simulink model "s_cd_ramp"  (R2016b)
(part 18 of 40)

      settings: AttributesFormatString=Latency = %<latency>
      mask Display:
      | port_label('input', 1, 'd');
      | port_label('output', 1, 'q');
      | disp(['Z^-', num2str(latency)]);
  pipeline69 : Subsystem  AncestorBlock=casper_library_delays/pipeline  mask(pipeline){latency=2}
      mask help:
      | An explicitly laid-out delay line to avoid mapping to SRL16s
      | for use in pipelining to help achieve timing closure.
      mask init:
      | pipeline_init(gcb,'latency',latency);
      settings: AttributesFormatString=Latency = %<latency>
      mask Display:
      | port_label('input', 1, 'd');
      | port_label('output', 1, 'q');
      | disp(['Z^-', num2str(latency)]);
  pipeline7 : Subsystem  AncestorBlock=casper_library_delays/pipeline  mask(pipeline){latency=2}
      mask help:
      | An explicitly laid-out delay line to avoid mapping to SRL16s
      | for use in pipelining to help achieve timing closure.
      mask init:
      | pipeline_init(gcb,'latency',latency);
      settings: AttributesFormatString=Latency = %<latency>
      mask Display:
      | port_label('input', 1, 'd');
      | port_label('output', 1, 'q');
      | disp(['Z^-', num2str(latency)]);
  pipeline70 : Subsystem  AncestorBlock=casper_library_delays/pipeline  mask(pipeline){latency=2}
      mask help:
      | An explicitly laid-out delay line to avoid mapping to SRL16s
      | for use in pipelining to help achieve timing closure.
      mask init:
      | pipeline_init(gcb,'latency',latency);
      settings: AttributesFormatString=Latency = %<latency>
      mask Display:
      | port_label('input', 1, 'd');
      | port_label('output', 1, 'q');
      | disp(['Z^-', num2str(latency)]);
  pipeline71 : Subsystem  AncestorBlock=casper_library_delays/pipeline  mask(pipeline){latency=2}
      mask help:
      | An explicitly laid-out delay line to avoid mapping to SRL16s
      | for use in pipelining to help achieve timing closure.
      mask init:
      | pipeline_init(gcb,'latency',latency);
      settings: AttributesFormatString=Latency = %<latency>
      mask Display:
      | port_label('input', 1, 'd');
      | port_label('output', 1, 'q');
      | disp(['Z^-', num2str(latency)]);
  pipeline72 : Subsystem  AncestorBlock=casper_library_delays/pipeline  mask(pipeline){latency=2}
      mask help:
      | An explicitly laid-out delay line to avoid mapping to SRL16s
      | for use in pipelining to help achieve timing closure.
      mask init:
      | pipeline_init(gcb,'latency',latency);
      settings: AttributesFormatString=Latency = %<latency>
      mask Display:
      | port_label('input', 1, 'd');
      | port_label('output', 1, 'q');
      | disp(['Z^-', num2str(latency)]);
  pipeline73 : Subsystem  AncestorBlock=casper_library_delays/pipeline  mask(pipeline){latency=2}
      mask help:
      | An explicitly laid-out delay line to avoid mapping to SRL16s
      | for use in pipelining to help achieve timing closure.
      mask init:
      | pipeline_init(gcb,'latency',latency);
      settings: AttributesFormatString=Latency = %<latency>
      mask Display:
      | port_label('input', 1, 'd');
      | port_label('output', 1, 'q');
      | disp(['Z^-', num2str(latency)]);
  pipeline74 : Subsystem  AncestorBlock=casper_library_delays/pipeline  mask(pipeline){latency=2}
      mask help:
      | An explicitly laid-out delay line to avoid mapping to SRL16s
      | for use in pipelining to help achieve timing closure.
      mask init:
      | pipeline_init(gcb,'latency',latency);
      settings: AttributesFormatString=Latency = %<latency>
      mask Display:
      | port_label('input', 1, 'd');
      | port_label('output', 1, 'q');
      | disp(['Z^-', num2str(latency)]);
  pipeline75 : Subsystem  AncestorBlock=casper_library_delays/pipeline  mask(pipeline){latency=2}
      mask help:
      | An explicitly laid-out delay line to avoid mapping to SRL16s
      | for use in pipelining to help achieve timing closure.
      mask init:
      | pipeline_init(gcb,'latency',latency);
      settings: AttributesFormatString=Latency = %<latency>
      mask Display:
      | port_label('input', 1, 'd');
      | port_label('output', 1, 'q');
      | disp(['Z^-', num2str(latency)]);
  pipeline76 : Subsystem  AncestorBlock=casper_library_delays/pipeline  mask(pipeline){latency=2}
      mask help:
      | An explicitly laid-out delay line to avoid mapping to SRL16s
      | for use in pipelining to help achieve timing closure.
      mask init:
      | pipeline_init(gcb,'latency',latency);
      settings: AttributesFormatString=Latency = %<latency>
      mask Display:
      | port_label('input', 1, 'd');
      | port_label('output', 1, 'q');
      | disp(['Z^-', num2str(latency)]);
  pipeline77 : Subsystem  AncestorBlock=casper_library_delays/pipeline  mask(pipeline){latency=2}
      mask help:
      | An explicitly laid-out delay line to avoid mapping to SRL16s
      | for use in pipelining to help achieve timing closure.
      mask init:
      | pipeline_init(gcb,'latency',latency);
      settings: AttributesFormatString=Latency = %<latency>
      mask Display:
      | port_label('input', 1, 'd');
      | port_label('output', 1, 'q');
      | disp(['Z^-', num2str(latency)]);
  pipeline78 : Subsystem  AncestorBlock=casper_library_delays/pipeline  mask(pipeline){latency=2}
      mask help:
      | An explicitly laid-out delay line to avoid mapping to SRL16s
      | for use in pipelining to help achieve timing closure.
      mask init:
      | pipeline_init(gcb,'latency',latency);
      settings: AttributesFormatString=Latency = %<latency>
      mask Display:
      | port_label('input', 1, 'd');
      | port_label('output', 1, 'q');
      | disp(['Z^-', num2str(latency)]);
  pipeline79 : Subsystem  AncestorBlock=casper_library_delays/pipeline  mask(pipeline){latency=2}
      mask help:
      | An explicitly laid-out delay line to avoid mapping to SRL16s
      | for use in pipelining to help achieve timing closure.
      mask init:
      | pipeline_init(gcb,'latency',latency);
      settings: AttributesFormatString=Latency = %<latency>
      mask Display:
      | port_label('input', 1, 'd');
      | port_label('output', 1, 'q');
      | disp(['Z^-', num2str(latency)]);
  pipeline8 : Subsystem  AncestorBlock=casper_library_delays/pipeline  mask(pipeline){latency=2}
      mask help:
      | An explicitly laid-out delay line to avoid mapping to SRL16s
      | for use in pipelining to help achieve timing closure.
      mask init:
      | pipeline_init(gcb,'latency',latency);
      settings: AttributesFormatString=Latency = %<latency>
      mask Display:
      | port_label('input', 1, 'd');
      | port_label('output', 1, 'q');
      | disp(['Z^-', num2str(latency)]);
  pipeline83 : Subsystem  AncestorBlock=casper_library_delays/pipeline  mask(pipeline){latency=2}
      mask help:
      | An explicitly laid-out delay line to avoid mapping to SRL16s
      | for use in pipelining to help achieve timing closure.
      mask init:
      | pipeline_init(gcb,'latency',latency);
      settings: AttributesFormatString=Latency = %<latency>
      mask Display:
      | port_label('input', 1, 'd');
      | port_label('output', 1, 'q');
      | disp(['Z^-', num2str(latency)]);
  pipeline84 : Subsystem  AncestorBlock=casper_library_delays/pipeline  mask(pipeline){latency=2}
      mask help:
      | An explicitly laid-out delay line to avoid mapping to SRL16s
      | for use in pipelining to help achieve timing closure.
      mask init:
      | pipeline_init(gcb,'latency',latency);
      settings: AttributesFormatString=Latency = %<latency>
      mask Display:
      | port_label('input', 1, 'd');
      | port_label('output', 1, 'q');
      | disp(['Z^-', num2str(latency)]);
  pipeline85 : Subsystem  AncestorBlock=casper_library_delays/pipeline  mask(pipeline){latency=2}
      mask help:
      | An explicitly laid-out delay line to avoid mapping to SRL16s
      | for use in pipelining to help achieve timing closure.
      mask init:
      | pipeline_init(gcb,'latency',latency);
      settings: AttributesFormatString=Latency = %<latency>
      mask Display:
      | port_label('input', 1, 'd');
      | port_label('output', 1, 'q');
      | disp(['Z^-', num2str(latency)]);
  pipeline86 : Subsystem  AncestorBlock=casper_library_delays/pipeline  mask(pipeline){latency=2}
      mask help:
      | An explicitly laid-out delay line to avoid mapping to SRL16s
      | for use in pipelining to help achieve timing closure.
      mask init:
      | pipeline_init(gcb,'latency',latency);
      settings: AttributesFormatString=Latency = %<latency>
      mask Display:
      | port_label('input', 1, 'd');
      | port_label('output', 1, 'q');
      | disp(['Z^-', num2str(latency)]);
  pipeline87 : Subsystem  AncestorBlock=casper_library_delays/pipeline  mask(pipeline){latency=2}
      mask help:
      | An explicitly laid-out delay line to avoid mapping to SRL16s
      | for use in pipelining to help achieve timing closure.
      mask init:
      | pipeline_init(gcb,'latency',latency);
      settings: AttributesFormatString=Latency = %<latency>
      mask Display:
      | port_label('input', 1, 'd');
      | port_label('output', 1, 'q');
      | disp(['Z^-', num2str(latency)]);
  pipeline88 : Subsystem  AncestorBlock=casper_library_delays/pipeline  mask(pipeline){latency=2}
      mask help:
      | An explicitly laid-out delay line to avoid mapping to SRL16s
      | for use in pipelining to help achieve timing closure.
      mask init:
      | pipeline_init(gcb,'latency',latency);
      settings: AttributesFormatString=Latency = %<latency>
      mask Display:
      | port_label('input', 1, 'd');
      | port_label('output', 1, 'q');
      | disp(['Z^-', num2str(latency)]);
  pipeline89 : Subsystem  AncestorBlock=casper_library_delays/pipeline  mask(pipeline){latency=2}
      mask help:
      | An explicitly laid-out delay line to avoid mapping to SRL16s
      | for use in pipelining to help achieve timing closure.
      mask init:
      | pipeline_init(gcb,'latency',latency);
      settings: AttributesFormatString=Latency = %<latency>
      mask Display:
      | port_label('input', 1, 'd');
      | port_label('output', 1, 'q');
      | disp(['Z^-', num2str(latency)]);
  pipeline9 : Subsystem  AncestorBlock=casper_library_delays/pipeline  mask(pipeline){latency=2}
      mask help:
      | An explicitly laid-out delay line to avoid mapping to SRL16s
      | for use in pipelining to help achieve timing closure.
      mask init:
      | pipeline_init(gcb,'latency',latency);
      settings: AttributesFormatString=Latency = %<latency>
      mask Display:
      | port_label('input', 1, 'd');
      | port_label('output', 1, 'q');
      | disp(['Z^-', num2str(latency)]);
  pipeline90 : Subsystem  AncestorBlock=casper_library_delays/pipeline  mask(pipeline){latency=2}
      mask help:
      | An explicitly laid-out delay line to avoid mapping to SRL16s
      | for use in pipelining to help achieve timing closure.
      mask init:
      | pipeline_init(gcb,'latency',latency);
      settings: AttributesFormatString=Latency = %<latency>
      mask Display:
      | port_label('input', 1, 'd');
      | port_label('output', 1, 'q');
      | disp(['Z^-', num2str(latency)]);
  pipeline91 : Subsystem  AncestorBlock=casper_library_delays/pipeline  mask(pipeline){latency=2}
      mask help:
      | An explicitly laid-out delay line to avoid mapping to SRL16s
      | for use in pipelining to help achieve timing closure.
      mask init:
      | pipeline_init(gcb,'latency',latency);
      settings: AttributesFormatString=Latency = %<latency>
      mask Display:
      | port_label('input', 1, 'd');
      | port_label('output', 1, 'q');
      | disp(['Z^-', num2str(latency)]);
  pipeline92 : Subsystem  AncestorBlock=casper_library_delays/pipeline  mask(pipeline){latency=1}
      mask help:
      | An explicitly laid-out delay line to avoid mapping to SRL16s
      | for use in pipelining to help achieve timing closure.
      mask init:
      | pipeline_init(gcb,'latency',latency);
      settings: AttributesFormatString=Latency = %<latency>
      mask Display:
      | port_label('input', 1, 'd');
      | port_label('output', 1, 'q');
      | disp(['Z^-', num2str(latency)]);
  pipeline93 : Subsystem  AncestorBlock=casper_library_delays/pipeline  mask(pipeline){latency=2}
      mask help:
      | An explicitly laid-out delay line to avoid mapping to SRL16s
      | for use in pipelining to help achieve timing closure.
      mask init:
      | pipeline_init(gcb,'latency',latency);
      settings: AttributesFormatString=Latency = %<latency>
      mask Display:
      | port_label('input', 1, 'd');
      | port_label('output', 1, 'q');
      | disp(['Z^-', num2str(latency)]);
  pipeline94 : Subsystem  AncestorBlock=casper_library_delays/pipeline  mask(pipeline){latency=2}
      mask help:
      | An explicitly laid-out delay line to avoid mapping to SRL16s
      | for use in pipelining to help achieve timing closure.
      mask init:
      | pipeline_init(gcb,'latency',latency);
      settings: AttributesFormatString=Latency = %<latency>
      mask Display:
      | port_label('input', 1, 'd');
      | port_label('output', 1, 'q');
      | disp(['Z^-', num2str(latency)]);
  pipeline95 : Subsystem  AncestorBlock=casper_library_delays/pipeline  mask(pipeline){latency=2}
      mask help:
      | An explicitly laid-out delay line to avoid mapping to SRL16s
      | for use in pipelining to help achieve timing closure.
      mask init:
      | pipeline_init(gcb,'latency',latency);
      settings: AttributesFormatString=Latency = %<latency>
      mask Display:
      | port_label('input', 1, 'd');
      | port_label('output', 1, 'q');
      | disp(['Z^-', num2str(latency)]);
  pipeline96 : Subsystem  AncestorBlock=casper_library_delays/pipeline  mask(pipeline){latency=2}
      mask help:
      | An explicitly laid-out delay line to avoid mapping to SRL16s
      | for use in pipelining to help achieve timing closure.
      mask init:
      | pipeline_init(gcb,'latency',latency);
      settings: AttributesFormatString=Latency = %<latency>
      mask Display:
      | port_label('input', 1, 'd');
      | port_label('output', 1, 'q');
      | disp(['Z^-', num2str(latency)]);
  qout : Subsystem  Tag=casper:bitsnap  AncestorBlock=casper_library_scopes/bitfield snapshot  mask(bitsnap){io_names=[d00 d01 d02 d03 d04 d05 d06 d07 dvalid sync], io_widths=[10 10 10 10 10 10 10 10 1 1], io_bps=[0 0 0 0 0 0 0 0 0 0], io_types=[0 0 0 0 0 0 0 0 2 2], show_format=on, snap_storage=bram, snap_dram_dimm=2, snap_dram_clock=250, snap_nsamples=11, snap_data_width=128, snap_offset=off, snap_circap=off, snap_value=off, snap_use_dsp48=off, snap_delay=0, extra_names=[c d], extra_widths=[30 2], extra_bps=[0 0], extra_types=[0 0]}
      mask prompts: io_names "Names [msb...lsb]"; io_widths "Bitwidths [msb...lsb]"; io_bps "Binary pts [msb...lsb]"; io_types "Data types [msb...lsb], ufix=0, fix=1, bool=2"; show_format "Print format string?"; snap_storage "Storage medium"; snap_dram_dimm "DRAM dimm"; snap_dram_clock "DRAM clock rate"; snap_nsamples "Number of Samples (2^?)"; snap_data_width "Data width"; snap_offset "Start delay support"; snap_circap "Circular capture support"; snap_value "Extra value capture support"; snap_use_dsp48 "Use DSP48s to implement counters"; snap_delay "Pre-snapshot delay"; extra_names "Names [msb...lsb]"; extra_widths "Widths [msb...lsb]"; extra_bps "Binary pts [msb...lsb]"; extra_types "Data types [msb...lsb], ufix=0, fix=1, bool=2"
      mask help:
      | A wrapped snapshot block. Allows specification of inputs to a snapblock word so the toolflow can automatically set up the scope.
      | See documentation for snapshot for explanation of parameters.
      mask init:
      | bitsnap_init(gcb);
      settings: AttributesFormatString=snap(10):uf10.0,uf10.0,uf10.0,uf10.0,uf10.0,uf10.0,uf10.0,uf10.0,b,b = 82 bits
      mask TypeOptions snap_storage: bram | dram
      mask Callback snap_storage: bitsnap_callback();
      mask TypeOptions snap_dram_dimm: 1 | 2 | 3 | 4
      mask TypeOptions snap_dram_clock: 200 | 250 | 266 | 300 | 333
      mask TypeOptions snap_data_width: 8 | 16 | 32 | 64 | 128
      mask Callback snap_value: bitsnap_callback();
  rdin_stall : xbsIndex_r4/Counter  cnt_type=Count Limited  cnt_to=1  operation=Up  start_count=0  cnt_by_val=1  arith_type=Unsigned  n_bits=1  bin_pt=0  load_pin=off  rst=off  en=on  explicit_period=on  period=1  use_behavioral_HDL=on  implementation=DSP48  use_rpm=off  dbl_ovrd=off  block_type=counter
  reord_dvalid_delay : xbsIndex_r4/Delay  rst=off  infoeditControl=Selection of Reset will increase slice count due to use of real FFs and instead of SRLs  en=off  latency=1  reg_retiming=on  dbl_ovrd=off  block_type=delay
      settings: infoedit=Hardware notes: A delay line is a chain, each link of which is an SRL16 or SRL32 followed by a flip-flop.
  reord_dvalid_delay2 : xbsIndex_r4/Delay  rst=off  infoeditControl=Selection of Reset will increase slice count due to use of real FFs and instead of SRLs  en=off  latency=3  reg_retiming=on  dbl_ovrd=off  block_type=delay
      settings: infoedit=Hardware notes: A delay line is a chain, each link of which is an SRL16 or SRL32 followed by a flip-flop.
  second : xbsIndex_r4/Delay  rst=off  infoeditControl=Selection of Reset will increase slice count due to use of real FFs and instead of SRLs  en=on  latency=1  reg_retiming=on  dbl_ovrd=off  block_type=delay
      settings: block_version=11.4
  sync_counter_en : Subsystem  Tag=xps:sw_reg  AncestorBlock=xps_library/software_register  mask(swreg){io_dir=From Processor, io_delay=0, sample_period=1, names=reg, bitwidths=1, bin_pts=0, arith_types=2, sim_port=off, show_format=on}
      mask prompts: io_dir "I/O direction"; io_delay "I/O delay"; sample_period "Sample period"; names "Bitfield names [msb...lsb]"; bitwidths "Bitfield widths"; bin_pts "Bitfield binary pts"; arith_types "Bitfield types, ufix=0, fix=1, bool=2"; sim_port "Provide sim input/output?"; show_format "Print format string?"
      mask help: A 32-bit software-accessible register. Can be divided into bitfields of varying widths and types using the fields in the block mask.
      mask init:
      | swreg_init(gcb)
      settings: AttributesFormatString=1input:b = 1 bits
      mask TypeOptions io_dir: To Processor | From Processor
      mask Callback io_dir:
      | mask_enables = get_param(gcb, 'MaskEnables');
      | mask_names = get_param(gcb, 'MaskNames');
      | if strcmp(get_param(gcb, 'io_dir'), 'To Processor'),
      |     mask_enables{ismember(mask_names, 'sample_period')} = 'off';
      | else
      |     mask_enables{ismember(mask_names, 'sample_period')} = 'on';
      | end
      | set_param(gcb, 'MaskEnables', mask_enables);
  sync_counter_rst : Subsystem  Tag=xps:sw_reg  AncestorBlock=xps_library/software_register  mask(swreg){io_dir=From Processor, io_delay=0, sample_period=1, names=reg, bitwidths=1, bin_pts=0, arith_types=2, sim_port=off, show_format=on}
      mask prompts: io_dir "I/O direction"; io_delay "I/O delay"; sample_period "Sample period"; names "Bitfield names [msb...lsb]"; bitwidths "Bitfield widths"; bin_pts "Bitfield binary pts"; arith_types "Bitfield types, ufix=0, fix=1, bool=2"; sim_port "Provide sim input/output?"; show_format "Print format string?"
      mask help: A 32-bit software-accessible register. Can be divided into bitfields of varying widths and types using the fields in the block mask.
      mask init:
      | swreg_init(gcb)
      settings: AttributesFormatString=1input:b = 1 bits
      mask TypeOptions io_dir: To Processor | From Processor
      mask Callback io_dir:
      | mask_enables = get_param(gcb, 'MaskEnables');
      | mask_names = get_param(gcb, 'MaskNames');
      | if strcmp(get_param(gcb, 'io_dir'), 'To Processor'),
      |     mask_enables{ismember(mask_names, 'sample_period')} = 'off';
      | else
      |     mask_enables{ismember(mask_names, 'sample_period')} = 'on';
      | end
      | set_param(gcb, 'MaskEnables', mask_enables);
  sync_delay1 : xbsIndex_r4/Delay  rst=off  infoeditControl=Selection of Reset will increase slice count due to use of real FFs and instead of SRLs  en=off  latency=3  reg_retiming=on  dbl_ovrd=off  block_type=delay
      settings: infoedit=Hardware notes: A delay line is a chain, each link of which is an SRL16 or SRL32 followed by a flip-flop.
  sync_delay2 : xbsIndex_r4/Delay  rst=off  infoeditControl=Selection of Reset will increase slice count due to use of real FFs and instead of SRLs  en=off  latency=3  reg_retiming=on  dbl_ovrd=off  block_type=delay
      settings: infoedit=Hardware notes: A delay line is a chain, each link of which is an SRL16 or SRL32 followed by a flip-flop.
  sync_delay{3..5,7..9} (6 alike) : xbsIndex_r4/Delay  rst=off  infoeditControl=Selection of Reset will increase slice count due to use of real FFs and instead of SRLs  en=off  latency=1  reg_retiming=on  dbl_ovrd=off  block_type=delay
      settings: infoedit=Hardware notes: A delay line is a chain, each link of which is an SRL16 or SRL32 followed by a flip-flop.
  sync_delay6 : xbsIndex_r4/Delay  rst=off  infoeditControl=Selection of Reset will increase slice count due to use of real FFs and instead of SRLs  en=off  latency=3  reg_retiming=on  dbl_ovrd=off  block_type=delay
      settings: infoedit=Hardware notes: A delay line is a chain, each link of which is an SRL16 or SRL32 followed by a flip-flop.
  sync_en_fifo : Subsystem  Tag=xps:sw_reg  AncestorBlock=xps_library/software_register  mask(swreg){io_dir=From Processor, io_delay=0, sample_period=1, names=reg, bitwidths=1, bin_pts=0, arith_types=2, sim_port=off, show_format=on}
      mask prompts: io_dir "I/O direction"; io_delay "I/O delay"; sample_period "Sample period"; names "Bitfield names [msb...lsb]"; bitwidths "Bitfield widths"; bin_pts "Bitfield binary pts"; arith_types "Bitfield types, ufix=0, fix=1, bool=2"; sim_port "Provide sim input/output?"; show_format "Print format string?"
      mask help: A 32-bit software-accessible register. Can be divided into bitfields of varying widths and types using the fields in the block mask.
      mask init:
      | swreg_init(gcb)
      settings: AttributesFormatString=1input:b = 1 bits
      mask TypeOptions io_dir: To Processor | From Processor
      mask Callback io_dir:
      | mask_enables = get_param(gcb, 'MaskEnables');
      | mask_names = get_param(gcb, 'MaskNames');
      | if strcmp(get_param(gcb, 'io_dir'), 'To Processor'),
      |     mask_enables{ismember(mask_names, 'sample_period')} = 'off';
      | else
      |     mask_enables{ismember(mask_names, 'sample_period')} = 'on';
      | end
      | set_param(gcb, 'MaskEnables', mask_enables);
  sync_en_qout : Subsystem  Tag=xps:sw_reg  AncestorBlock=xps_library/software_register  mask(swreg){io_dir=From Processor, io_delay=0, sample_period=1, names=reg, bitwidths=1, bin_pts=0, arith_types=2, sim_port=off, show_format=on}
      mask prompts: io_dir "I/O direction"; io_delay "I/O delay"; sample_period "Sample period"; names "Bitfield names [msb...lsb]"; bitwidths "Bitfield widths"; bin_pts "Bitfield binary pts"; arith_types "Bitfield types, ufix=0, fix=1, bool=2"; sim_port "Provide sim input/output?"; show_format "Print format string?"
      mask help: A 32-bit software-accessible register. Can be divided into bitfields of varying widths and types using the fields in the block mask.
      mask init:
      | swreg_init(gcb)
      settings: AttributesFormatString=1input:b = 1 bits
      mask TypeOptions io_dir: To Processor | From Processor
      mask Callback io_dir:
      | mask_enables = get_param(gcb, 'MaskEnables');
      | mask_names = get_param(gcb, 'MaskNames');
      | if strcmp(get_param(gcb, 'io_dir'), 'To Processor'),
      |     mask_enables{ismember(mask_names, 'sample_period')} = 'off';
      | else
      |     mask_enables{ismember(mask_names, 'sample_period')} = 'on';
      | end
      | set_param(gcb, 'MaskEnables', mask_enables);
  sync_en_reord : Subsystem  Tag=xps:sw_reg  AncestorBlock=xps_library/software_register  mask(swreg){io_dir=From Processor, io_delay=0, sample_period=1, names=reg, bitwidths=1, bin_pts=0, arith_types=2, sim_port=off, show_format=on}
      mask prompts: io_dir "I/O direction"; io_delay "I/O delay"; sample_period "Sample period"; names "Bitfield names [msb...lsb]"; bitwidths "Bitfield widths"; bin_pts "Bitfield binary pts"; arith_types "Bitfield types, ufix=0, fix=1, bool=2"; sim_port "Provide sim input/output?"; show_format "Print format string?"
      mask help: A 32-bit software-accessible register. Can be divided into bitfields of varying widths and types using the fields in the block mask.
      mask init:
      | swreg_init(gcb)
      settings: AttributesFormatString=1input:b = 1 bits
      mask TypeOptions io_dir: To Processor | From Processor
      mask Callback io_dir:
      | mask_enables = get_param(gcb, 'MaskEnables');
      | mask_names = get_param(gcb, 'MaskNames');
      | if strcmp(get_param(gcb, 'io_dir'), 'To Processor'),
      |     mask_enables{ismember(mask_names, 'sample_period')} = 'off';
      | else
      |     mask_enables{ismember(mask_names, 'sample_period')} = 'on';
      | end
      | set_param(gcb, 'MaskEnables', mask_enables);
  tag_stall : xbsIndex_r4/Counter  cnt_type=Count Limited  cnt_to=1  operation=Up  start_count=0  cnt_by_val=1  arith_type=Unsigned  n_bits=1  bin_pt=0  load_pin=off  rst=off  en=on  explicit_period=on  period=1  use_behavioral_HDL=on  implementation=DSP48  use_rpm=off  dbl_ovrd=off  block_type=counter
  wrin_stall : xbsIndex_r4/Counter  cnt_type=Count Limited  cnt_to=1  operation=Up  start_count=0  cnt_by_val=1  arith_type=Unsigned  n_bits=1  bin_pt=0  load_pin=off  rst=off  en=on  explicit_period=on  period=1  use_behavioral_HDL=on  implementation=DSP48  use_rpm=off  dbl_ovrd=off  block_type=counter
  sync_out : Outport
  q : Outport  Port=2
  dv : Outport  Port=3
  hmc_error : Outport  Port=4
  parity_error : Outport  Port=5
  misco : Outport  Port=6
  tag scope: sync_trig=global
  wires:
  Logical6/1 -> Logical7/2, Delay68/1
  Delay44/1 -> Delay66/1, Logical7/1
  Delay37/1 -> Delay36/1, Logical4/2
  Delay31/1 -> Logical6/1
  Delay15/1 -> Delay31/1
  Logical5/1 -> Delay44/1
  Logical7/1 -> Delay45/1
  Delay14/1 -> Logical5/1, Delay54/1
  Inverter/1 -> Logical4/1
  Logical4/1 -> Delay14/3, Delay14/1
  Delay43/1 -> Logical6/2
  Delay11/1 -> [hmc_sync], Gateway Out8/1
  pipeline1/1(q) -> Delay37/1, Delay47/1
  Delay45/1 -> Delay11/1
  Gateway Out9/1 -> Scope1/1
  Gateway Out15/1 -> Scope1/7
  Gateway Out16/1 -> Scope1/8
  Gateway Out17/1 -> Scope1/9
  Gateway Out14/1 -> Scope1/6
  Gateway Out11/1 -> Scope1/3
  Gateway Out10/1 -> Scope1/2
  Gateway Out12/1 -> Scope1/4
  Gateway Out13/1 -> Scope1/5
  Gateway Out18/1 -> Scope1/10
  Reinterpret2/1 -> Gateway Out18/1
  Slice6/1 -> Reinterpret2/1
  Reinterpret1/1 -> Delay41/1
  Slice5/1 -> Reinterpret1/1
  Delay68/1 -> Delay67/1
  Delay67/1 -> Gateway Out15/1
  Delay66/1 -> Delay65/1
  Delay65/1 -> Gateway Out14/1
  Delay64/1 -> Delay53/1
  Delay5/1 -> Delay9/1
  Delay63/1 -> Delay64/1
  Delay41/1 -> Delay42/1
  Delay42/1 -> Delay46/1
  Delay46/1 -> Delay52/1
  [dout] -> Slice5/1
  Delay40/1 -> Delay39/1
  Delay48/1 -> Delay50/1, Gateway Out7/1
  Delay59/1 -> Gateway Out13/1
  Delay58/1 -> Gateway Out12/1
  Delay57/1 -> Gateway Out11/1
  Delay56/1 -> Gateway Out10/1
  Delay55/1 -> Gateway Out9/1
  Delay54/1 -> Delay59/1
  Delay53/1 -> Delay58/1
  Delay52/1 -> Delay57/1
  Delay51/1 -> Delay56/1
  Delay50/1 -> Delay55/1
  Delay47/1 -> Delay38/1
  Delay49/1 -> Delay51/1
  Delay39/1 -> Delay49/1
  Delay38/1 -> Delay48/1
  Delay36/1 -> Delay43/1
  Gateway Out8/1 -> Scope/9
  Delay35/1 -> Gateway Out5/1
  Delay34/1 -> Gateway Out/1
  Delay33/1 -> Delay34/1
  Delay32/1 -> Delay33/1
  Gateway Out7/1 -> Scope/8
  Delay30/1 -> pipeline8/1(d)
  Delay29/1 -> pipeline7/1(d)
  Delay28/1 -> pipeline6/1(d)
  Delay27/1 -> AddSub/1
  Delay26/1 -> Gateway Out6/1
  Gateway Out6/1 -> Scope/7
  Gateway Out5/1 -> Scope/6
  [rin] -> Gateway Out4/1
  [win] -> Gateway Out3/1
  [wadd] -> Gateway Out2/1
  [lsb] -> Delay32/1
  Reinterpret/1 -> Gateway Out1/1
  Slice4/1 -> Reinterpret/1
  [din] -> Slice4/1
  Gateway Out4/1 -> Scope/5
  Delay3/1 -> pipeline161/1(d), Delay14/2, Logical5/2
  second/1 -> pipeline162/1(d)
  AddSub/1 -> pipeline159/1(d)  "rd_add_HR"
  Gateway Out3/1 -> Scope/4
  Gateway Out2/1 -> Scope/3
  Gateway Out1/1 -> Scope/2
  Gateway Out/1 -> Scope/1
  Delay16/1 -> Delay17/1
  Delay21/1 -> Delay16/1
  misci/1 -> Delay21/1
  pipeline14/1(q) -> Delay8/1
  delay/1 -> pipeline14/1(d)  "delay"
  Delay13/1 -> second/1
  pipeline10/1(q) -> [dout]
  [rin] -> rdin_stall/1
  [win] -> wrin_stall/1
  [wadd] -> Delay73/1
  Delay10/1 -> second/2
  [din] -> parity_generation0/1(din)
  Slice1/1 -> [lsb]
  d/1 -> pipeline10/1(d)  "d_in"
  [dout] -> Delay13/1
  sync/1 -> pipeline13/1(d), pipeline15/1(d), pipeline1/1(d)  "sync_in"
  en/1 -> pipeline12/1(d), pipeline11/1(d), pipeline9/1(d)  "en_in"
  pipeline9/1(q) -> addr_stall/2, Delay40/1  "en"
  pipeline12/1(q) -> Delay10/1
  pipeline6/1(q) -> [hmc_rin]
  pipeline7/1(q) -> [hmc_win]
  parity_generation0/1(dout) -> Delay25/1  "reg_din"
  [hmc_din_256] -> pipeline4/1(d)
  pipeline8/1(q) -> [hmc_waddr]
  [hmc_waddr] -> pipeline3/1(d)
  [hmc_raddr] -> pipeline5/1(d)
  pipeline16/1(q) -> Gateway Out28/1, hmc/6, Register5/1  "hmc_tag_in"
  [hmc_tag] -> pipeline16/1(d)
  [hmc_win] -> pipeline18/1(d)
  [hmc_rin] -> pipeline17/1(d)
  pipeline19/1(q) -> Delay80/1  "hmc_dout"
  pipeline20/1(q) -> Delay79/1, Convert12/1, Convert13/1  "hmc_dvalid"
  pipeline23/1(q) -> Delay76/1  "rd_ready"
  pipeline24/1(q) -> Delay71/1  "init_done"
  pipeline25/1(q) -> Delay69/1  "post_ok"
  Logical1/1 -> delay20/1
  [hmc_reord_data] -> Slice3/1
  parity_check0/1(dout) -> [hmc_parity_data0]
  [hmc_dvalid] -> Gateway Out17/1
  Convert1/1 -> [hmc_dvalid]
  parity_check0/2(error) -> Delay74/1
  Delay1/1 -> [hmc_delay], Delay26/1, AddSub/2
  Delay22/1 -> pipeline2/1(d)
  pipeline2/1(q) -> [hmc_raddr]
  pipeline11/1(q) -> Delay24/1
  addr/1 -> Delay23/1  "addr"
  Delay4/1 -> Delay12/1, Delay27/1
  Delay2/1 -> pipeline160/1(d), Delay35/1
  Delay12/1 -> Delay2/1
  Delay9/1 -> Delay3/1, Delay15/1, Inverter/1, Delay63/1
  Delay8/1 -> Delay1/1
  Delay23/1 -> Delay4/1, Slice1/1
  Delay24/1 -> Delay5/1
  pipeline21/1(q) -> Relational2/1, Relational3/1, Delay78/1  "hmc_tag_out"
  pipeline22/1(q) -> Delay77/1  "wr_ready"
  Constant/1 -> AddSub1/2
  cd_hmc_rd_tag_err/1(sim_out) -> To Workspace1/1
  AddSub1/1 -> Relational/2  "tp4"
  [hmc_din] -> Delay60/1, Concat/1
  addr_stall/1 -> Convert2/1  "stall"
  pipeline13/1(q) -> addr_stall/1
  Convert2/1 -> addr/2
  pipeline15/1(q) -> addr/1
  tag_stall/1 -> Delay70/1
  [rin] -> Delay75/1
  Slice3/1 -> parity_check0/2(din)
  [hmc_reord_dvalid] -> parity_check0/1(en)
  [hmc_reord_data] -> Slice7/1
  Slice7/1 -> parity_check1/2(din)
  [hmc_reord_dvalid] -> parity_check1/1(en)
  parity_check1/2(error) -> Delay61/1
  Logical2/1 -> sync_delay2/1
  Delay74/1 -> Logical2/1
  Delay61/1 -> Logical2/2
  parity_check1/1(dout) -> [hmc_parity_data1]
  [radd] -> Delay72/1
  Concat/1 -> [hmc_din_256]
  rdin_stall/1 -> Convert5/1
  wrin_stall/1 -> Convert6/1
  Convert5/1 -> Delay28/1
  Convert6/1 -> Delay29/1
  [hmc_parity_data0] -> FIFO0/1
  cd_hmc_fifo_full/1(sim_out) -> To Workspace2/1
  FIFO1/4 -> [fifo1_full]
  FIFO0/4 -> [fifo0_full]
  [fifo0_full] -> Logical3/1
  [fifo1_full] -> Logical3/2
  cd_hmc_fifo_empty/1(sim_out) -> To Workspace3/1
  [fifo0_empty] -> Logical8/1
  [fifo1_empty] -> Logical8/2
  FIFO0/2 -> [fifo0_empty]
  FIFO1/2 -> [fifo1_empty]
  Relational/1 -> edge_detect5/1, Gateway Out34/1, cd_hmc_rd_tag_err/1(out_error)  "cd_hmc_rd_tag_err"
  [hmc_parity_data0] -> Slice6/1
  Delay72/1 -> Delay22/1
  Delay73/1 -> Delay30/1
  Delay75/1 -> tag_stall/1
  [hmc_tag_out] -> Register/1  "tp1"
  Register/1 -> Relational/1, AddSub1/1  "tp3"
  [hmc_dvalid] -> AddSub1/3, Register/2, Delay62/1  "tp2"
  Mux/1 -> pipeline115/1(d)  "Q"
  delay9/1 -> delay6/1  "dv_tp2"
  sync_delay2/1 -> sync_delay3/1
  sync_delay3/1 -> pipeline116/1(d)
  delay4/1 -> delay5/1
  delay5/1 -> pipeline114/1(d)
  delay6/1 -> pipeline113/1(d)  "dvalid"
  sync_delay8/1 -> Convert7/1  "sync"
  sync_delay1/1 -> sync_delay4/1
  delay10/1 -> sync_delay7/1
  Counter1/1 -> [hmc_tag]  "hmc_tag_gen"
  Delay62/1 -> Relational/3  "tp6"
  Constant2/1 -> HMC_reord_bram/5
  Constant3/1 -> HMC_reord_bram/6
  HMC_reord_bram/1 -> Terminator35/1
  reord_dvalid_delay/1 -> reord_dvalid_delay2/1
  Delay60/1 -> Concat/2
  Convert3/1 -> Counter1/1
  Delay70/1 -> Convert3/1
  Reorder_cntrl/2(bram_rd_en) -> HMC_reord_bram/7, Gateway Out36/1, reord_dvalid_delay/1
  delay7/1 -> pipeline112/1(d)
  cd_hmc_post/1(sim_out) -> To Workspace10/1
  Register2/1 -> cd_hmc_fifo_full/1(out_full)
  Logical3/1 -> Register2/3, Register2/1
  Register3/1 -> cd_hmc_fifo_empty/1(out_empty)
  Logical8/1 -> Register3/3, Register3/1
  [hmc_post] -> cd_hmc_post/1(out_post), edge_detect2/1
  [hmc_sync] -> Register2/2
  [hmc_sync] -> Register3/2
  [hmc_reord_dvalid] -> edge_detect/1(in)
  delay17/1 -> delay7/1
  delay18/1 -> delay17/1
  delay19/1 -> delay18/1
  delay20/1 -> delay21/1
  delay21/1 -> delay22/1
  delay22/1 -> delay23/1
  delay23/1 -> delay19/1
  [hmc_dout] -> Slice18/1
  [hmc_reord_sync] -> edge_detect1/1
  Convert7/1 -> pipeline117/1(d)
  edge_detect1/1 -> sync_delay1/1
  sync_delay4/1 -> sync_delay5/1, Gateway Out16/1
  sync_delay5/1 -> sync_delay6/1
  sync_delay6/1 -> sync_delay8/1
  delay24/1 -> delay9/1
  delay25/1 -> delay24/1
  [hmc_parity_data1] -> FIFO1/1
  delay27/1 -> delay25/1
  edge_detect/1(out) -> delay11/1
  delay11/1 -> delay27/1
  Slice17/1 -> Convert8/1
  Convert8/1 -> [hmc_reord_sync]
  Concat2/1 -> HMC_reord_bram/2
  Slice18/1 -> Concat2/2
  HMC_reord_bram/2 -> Slice10/1, Slice17/1
  [hmc_sync] -> Register5/2, pipeline27/1(d)  "hmc_sync"
  pipeline27/1(q) -> Register5/3
  Register5/1 -> Relational2/2
  Relational2/1 -> Inverter4/1, edge_detect3/1
  Inverter4/1 -> Logical11/2
  Delay69/1 -> Delay84/1
  Delay71/1 -> Delay86/1
  Delay76/1 -> [hmc_rd_rdy]
  Delay77/1 -> [hmc_wr_ready]
  Delay78/1 -> [hmc_tag_out]
  Delay79/1 -> Convert1/1
  Delay80/1 -> [hmc_dout]
  edge_detect3/1 -> [hmc_sync_regen]
  [hmc_sync_regen] -> Concat2/1
  Concat1/1 -> [hmc_reord_data]
  Constant1/1 -> Concat1/1
  Slice10/1 -> Concat1/2
  Gateway Out34/1 -> To Workspace20/1
  Delay17/1 -> pipeline163/1(d)
  Delay25/1 -> Convert/1
  [hmc_tag] -> pipeline28/1(d)
  pipeline28/1(q) -> Register7/1
  Slice/1 -> Convert10/1, Delay82/1
  Delay82/1 -> Convert9/1
  Register7/1 -> Relational3/2
  Logical9/1 -> Relational3/3
  Inverter5/1 -> Logical9/2
  Relational3/1 -> Inverter5/1, Register8/3
  Register6/1 -> Register8/1
  Delay81/1 -> pipeline29/1(d)
  pipeline29/1(q) -> Slice/1, Delay83/1
  Convert9/1 -> Register7/3, Register6/3
  Convert10/1 -> Register9/2, Register8/2, Register7/2, Register6/2
  Delay83/1 -> Register6/1
  Gateway Out19/1 -> To Workspace4/1
  Gateway Out21/1 -> To Workspace6/1
  Register8/1 -> Register9/1
  [hmc_reord_dvalid] -> Register9/3
  Register9/1 -> delay10/1
  sync_delay7/1 -> sync_delay9/1
  sync_delay9/1 -> delay4/1
  cd_hmc_post_counter/1(sim_out) -> To Workspace12/1
  Counter2/1 -> cd_hmc_post_counter/1(out_counter)
  cd_hmc_rd_tag_counter/1(sim_out) -> To Workspace13/1
  Counter3/1 -> cd_hmc_rd_tag_counter/1(out_counter)
  [hmc_sync] -> Counter3/1
  Logical11/1 -> Relational2/3
  Convert12/1 -> Logical11/1
  Convert13/1 -> Logical9/1
  cd_hmc_fifo1_level/1(sim_out) -> To Workspace14/1
  cd_hmc_fifo0_level/1(sim_out) -> To Workspace15/1
  Delay84/1 -> Delay85/1
  Delay85/1 -> [hmc_post]
  Delay86/1 -> Delay87/1
  Delay87/1 -> [hmc_init]
  cd_hmc_init/1(sim_out) -> To Workspace16/1
  [hmc_init] -> cd_hmc_init/1(out_init), edge_detect4/1
  cd_hmc_init_counter/1(sim_out) -> To Workspace17/1
  Counter4/1 -> cd_hmc_init_counter/1(out_counter)
  [hmc_sync] -> Counter2/1
  [hmc_sync] -> Counter4/1
  [hmc_init] -> Inverter2/1
  [hmc_post] -> Inverter6/1
  Inverter2/1 -> Logical1/1
  Inverter6/1 -> Logical1/2
  Constant9/1 -> pipeline171/1(d)
  Constant8/1 -> pipeline172/1(d)
  hmc/11 -> pipeline24/1(d)
  hmc/12 -> pipeline25/1(d)
  hmc/10 -> Terminator7/1
  hmc/9 -> Terminator6/1
  hmc/8 -> Terminator5/1
  hmc/7 -> Terminator3/1
  hmc/6 -> Terminator2/1
  hmc/5 -> pipeline21/1(d)
  hmc/4 -> pipeline23/1(d)
  hmc/3 -> pipeline22/1(d)
  hmc/2 -> pipeline20/1(d)
  hmc/1 -> pipeline19/1(d)
  Constant6/1 -> pipeline170/1(d)
  Constant5/1 -> pipeline169/1(d)
  Constant10/1 -> pipeline168/1(d)
  Constant7/1 -> pipeline167/1(d)
  pipeline5/1(q) -> Gateway Out27/1, hmc/5  "hmc_rdadd"
  pipeline17/1(q) -> Gateway Out26/1, hmc/4  "hmc_rin"
  pipeline4/1(q) -> hmc/3  "hmc_din"
  pipeline3/1(q) -> Gateway Out24/1, hmc/2  "hmc_wadd"
  pipeline18/1(q) -> Gateway Out25/1, hmc/1  "hmc_win"
  pipeline112/1(q) -> hmc_error/1
  pipeline114/1(q) -> misco/1
  pipeline115/1(q) -> q/1, [q_out]
  pipeline116/1(q) -> parity_error/1
  pipeline117/1(q) -> [q_sync], Gateway Out19/1, sync_out/1
  edge_detect2/1 -> Counter2/2
  edge_detect4/1 -> Counter4/2
  edge_detect5/1 -> Counter3/2
  Convert/1 -> [hmc_din]
  pipeline47/1(q) -> edge_detect7/1
  edge_detect7/1 -> [sync_trig]
  Gateway Out24/1 -> To Workspace9/1
  Gateway Out25/1 -> To Workspace11/1
  Gateway Out26/1 -> To Workspace18/1
  Gateway Out27/1 -> To Workspace19/1
  Gateway Out28/1 -> To Workspace21/1
  pipeline133/1(q) -> Counter5/1
  pipeline134/1(q) -> Counter5/2
  sync_counter_en/1(in_reg) -> pipeline134/1(d)
  sync_counter_rst/1(in_reg) -> pipeline133/1(d)
  Counter5/1 -> pipeline135/1(d)
  Relational4/1 -> pipeline47/1(d)
  Constant11/1 -> pipeline136/1(d)
  pipeline135/1(q) -> Relational4/1
  pipeline136/1(q) -> Relational4/2
  bus_expand5/1(msb_out8) -> pipeline120/1(d)  "hmc_out1"
  bus_expand5/8(lsb_out1) -> pipeline127/1(d)  "hmc_out8"
  Slice14/1 -> bus_expand5/1(bus_in)
  bus_expand8/1(msb_out8) -> pipeline103/1(d)  "hmc_out9"
  bus_expand8/8(lsb_out1) -> pipeline119/1(d)  "hmc_out16"
  Slice15/1 -> bus_expand8/1(bus_in)
  [hmc_reord_data] -> pipeline141/1(d), pipeline142/1(d)
  [hmc_reord_dvalid] -> pipeline139/1(d)
  [hmc_reord_sync] -> pipeline140/1(d)
  pipeline120/1(q) -> hmc_reord0/1(in_d00)
  pipeline121/1(q) -> hmc_reord0/2(in_d01)
  pipeline122/1(q) -> hmc_reord0/3(in_d02)
  pipeline124/1(q) -> hmc_reord0/5(in_d04)
  pipeline125/1(q) -> hmc_reord0/6(in_d05)
  pipeline126/1(q) -> hmc_reord0/7(in_d06)
  pipeline128/1(q) -> hmc_reord0/9(we)
  pipeline137/1(q) -> hmc_reord0/10(trig)
  pipeline119/1(q) -> hmc_reord1/8(in_d07)
  pipeline118/1(q) -> hmc_reord1/7(in_d06)
  pipeline111/1(q) -> hmc_reord1/6(in_d05)
  pipeline107/1(q) -> hmc_reord1/5(in_d04)
  pipeline106/1(q) -> hmc_reord1/4(in_d03)
  pipeline105/1(q) -> hmc_reord1/3(in_d02)
  pipeline104/1(q) -> hmc_reord1/2(in_d01)
  pipeline103/1(q) -> hmc_reord1/1(in_d00)
  bus_expand5/2(out7) -> pipeline121/1(d)
  bus_expand5/4(out5) -> pipeline123/1(d)
  bus_expand5/7(out2) -> pipeline126/1(d)
  bus_expand5/3(out6) -> pipeline122/1(d)
  bus_expand8/7(out2) -> pipeline118/1(d)
  bus_expand5/5(out4) -> pipeline124/1(d)
  bus_expand5/6(out3) -> pipeline125/1(d)
  bus_expand8/5(out4) -> pipeline107/1(d)
  bus_expand8/4(out5) -> pipeline106/1(d)
  bus_expand8/6(out3) -> pipeline111/1(d)
  bus_expand8/3(out6) -> pipeline105/1(d)
  bus_expand8/2(out7) -> pipeline104/1(d)
  pipeline139/1(q) -> pipeline128/1(d)
  pipeline141/1(q) -> Slice14/1
  pipeline142/1(q) -> Slice15/1
  [sync_trig] -> Logical17/2
  Logical17/1 -> pipeline137/1(d)
  sync_en_reord/1(in_reg) -> pipeline144/1(d), pipeline138/1(d)
  pipeline138/1(q) -> Logical22/2
  pipeline140/1(q) -> Logical22/1
  Logical22/1 -> edge_detect6/1(in)
  pipeline127/1(q) -> hmc_reord0/8(in_d07)
  pipeline123/1(q) -> hmc_reord0/4(in_d03)
  edge_detect6/1(out) -> Logical17/1
  pipeline143/1(q) -> pipeline150/1(d)
  [sync_trig] -> Logical25/2
  edge_detect10/1(out) -> Logical25/1
  Logical25/1 -> pipeline149/1(d)
  Logical26/1 -> edge_detect10/1(in)
  pipeline144/1(q) -> Logical26/2
  pipeline145/1(q) -> Logical26/1
  [hmc_reord_sync] -> pipeline145/1(d)
  [hmc_reord_dvalid] -> pipeline143/1(d)
  [hmc_tag_out] -> Gateway Out81/1, HMC_reord_bram/1
  pipeline149/1(q) -> hmc_reord1/10(trig)
  pipeline150/1(q) -> hmc_reord1/9(we)
  [hmc_dvalid] -> Gateway Out82/1, HMC_reord_bram/3
  Counter6/1 -> pipeline157/1(d)
  Constant12/1 -> Relational5/2
  [hmc_win] -> Gateway Out35/1, Counter7/2
  Register4/1 -> pipeline156/1(d)
  data_in_counter/1(sim_out) -> To Workspace25/1
  Counter8/1 -> pipeline158/1(d)
  Constant13/1 -> Relational6/2
  [hmc_dvalid] -> Counter9/2
  Register10/1 -> pipeline155/1(d)
  data_out_counter/1(sim_out) -> To Workspace26/1
  Gateway Out29/1 -> To Workspace22/1
  Gateway Out30/1 -> To Workspace23/1
  Gateway Out31/1 -> To Workspace24/1
  Gateway Out32/1 -> To Workspace27/1
  Gateway Out33/1 -> To Workspace28/1
  Gateway Out35/1 -> To Workspace29/1
  Relational5/1 -> pipeline153/1(d), Register4/2, Gateway Out30/1, Counter7/1
  pipeline61/1(q) -> Register10/3
  Relational6/1 -> pipeline61/1(d), Register10/2, Counter9/1
  Counter9/1 -> pipeline152/1(d)
  Counter7/1 -> pipeline154/1(d)
  pipeline152/1(q) -> Register10/1
  pipeline153/1(q) -> Gateway Out33/1, Register4/3
  pipeline154/1(q) -> Gateway Out31/1, Register4/1
  pipeline155/1(q) -> data_out_counter/1(out_counter)
  pipeline156/1(q) -> Gateway Out32/1, data_in_counter/1(out_counter)
  pipeline157/1(q) -> Gateway Out29/1, Relational5/1
  pipeline158/1(q) -> Relational6/1
  pipeline159/1(q) -> [radd]
  pipeline160/1(q) -> [wadd]
  pipeline161/1(q) -> [rin], [win]
  pipeline162/1(q) -> [din]
  pipeline163/1(q) -> Delay81/1
  [hmc_sync_regen] -> Reorder_cntrl/1(rst)
  [hmc_tag_out] -> Reorder_cntrl/2(tag)
  [hmc_dvalid] -> Reorder_cntrl/3(dvalid)
  Reorder_cntrl/1(bram_rd_addr) -> Gateway Out23/1, HMC_reord_bram/4
  Gateway Out23/1 -> To Workspace8/1
  Gateway Out36/1 -> To Workspace30/1
  pipeline167/1(q) -> hmc/7
  pipeline168/1(q) -> hmc/8
  pipeline169/1(q) -> hmc/9
  pipeline170/1(q) -> hmc/10
  pipeline171/1(q) -> hmc/11
  pipeline172/1(q) -> hmc/12
  [hmc_parity_data0] -> bus_expand9/1(bus_in)
  [hmc_parity_data1] -> bus_expand10/1(bus_in)
  Gateway Out43/1 -> To Workspace37/1
  bus_expand9/1(msb_out8) -> Gateway Out43/1
  Gateway Out45/1 -> To Workspace39/1
  Gateway Out46/1 -> To Workspace40/1
  Gateway Out47/1 -> To Workspace41/1
  Gateway Out48/1 -> To Workspace42/1
  bus_expand9/5(out4) -> Gateway Out48/1
  Gateway Out49/1 -> To Workspace43/1
  bus_expand9/6(out3) -> Gateway Out49/1
  Gateway Out50/1 -> To Workspace44/1
  bus_expand9/7(out2) -> Gateway Out50/1
  Gateway Out51/1 -> To Workspace45/1
  bus_expand9/4(out5) -> Gateway Out47/1
  bus_expand9/3(out6) -> Gateway Out46/1
  bus_expand9/2(out7) -> Gateway Out45/1
  bus_expand9/8(lsb_out1) -> Gateway Out51/1
  Gateway Out52/1 -> To Workspace46/1
  bus_expand10/1(msb_out8) -> Gateway Out52/1
  bus_expand10/2(out7) -> Gateway Out53/1
  bus_expand10/3(out6) -> Gateway Out54/1
  bus_expand10/4(out5) -> Gateway Out55/1
  bus_expand10/5(out4) -> Gateway Out56/1
  bus_expand10/6(out3) -> Gateway Out57/1
  bus_expand10/7(out2) -> Gateway Out58/1
  bus_expand10/8(lsb_out1) -> Gateway Out59/1
  Gateway Out54/1 -> To Workspace47/1
  Gateway Out55/1 -> To Workspace48/1
  Gateway Out56/1 -> To Workspace49/1
  Gateway Out57/1 -> To Workspace50/1
  Gateway Out58/1 -> To Workspace51/1
  Gateway Out59/1 -> To Workspace52/1
  Gateway Out53/1 -> To Workspace38/1
  bus_expand12/1(msb_out8) -> Gateway Out40/1
  bus_expand12/5(out4) -> Gateway Out61/1
  bus_expand12/6(out3) -> Gateway Out62/1
  bus_expand12/7(out2) -> Gateway Out63/1
  bus_expand12/4(out5) -> Gateway Out60/1
  bus_expand12/3(out6) -> Gateway Out44/1
  bus_expand12/2(out7) -> Gateway Out41/1
  bus_expand12/8(lsb_out1) -> Gateway Out64/1
  bus_expand11/1(msb_out8) -> Gateway Out65/1
  bus_expand11/2(out7) -> Gateway Out66/1
  bus_expand11/3(out6) -> Gateway Out67/1
  bus_expand11/4(out5) -> Gateway Out68/1
  bus_expand11/5(out4) -> Gateway Out69/1
  bus_expand11/6(out3) -> Gateway Out70/1
  bus_expand11/7(out2) -> Gateway Out71/1
  bus_expand11/8(lsb_out1) -> Gateway Out72/1
  Gateway Out72/1 -> To Workspace66/1
  Gateway Out71/1 -> To Workspace65/1
  Gateway Out70/1 -> To Workspace64/1
  Gateway Out69/1 -> To Workspace63/1
  Gateway Out68/1 -> To Workspace62/1
  Gateway Out67/1 -> To Workspace61/1
  Gateway Out66/1 -> To Workspace35/1
  Gateway Out65/1 -> To Workspace60/1
  Gateway Out63/1 -> To Workspace58/1
  Gateway Out64/1 -> To Workspace59/1
  Gateway Out62/1 -> To Workspace57/1
  Gateway Out61/1 -> To Workspace56/1
  Gateway Out60/1 -> To Workspace55/1
  Gateway Out44/1 -> To Workspace54/1
  Gateway Out41/1 -> To Workspace53/1
  Gateway Out40/1 -> To Workspace34/1
  bus_expand13/2(out7) -> Gateway Out73/1
  bus_expand13/3(out6) -> Gateway Out74/1
  bus_expand13/4(out5) -> Gateway Out75/1
  bus_expand13/5(out4) -> Gateway Out76/1
  bus_expand13/6(out3) -> Gateway Out77/1
  bus_expand13/7(out2) -> Gateway Out78/1
  bus_expand13/8(lsb_out1) -> Gateway Out79/1
  Gateway Out79/1 -> To Workspace74/1
  Gateway Out78/1 -> To Workspace73/1
  Gateway Out77/1 -> To Workspace72/1
  Gateway Out76/1 -> To Workspace71/1
  Gateway Out75/1 -> To Workspace70/1
  Gateway Out74/1 -> To Workspace69/1
  Gateway Out73/1 -> To Workspace67/1
  [q_out] -> bus_expand13/1(bus_in)
  bus_expand13/1(msb_out8) -> Gateway Out80/1
  Gateway Out80/1 -> To Workspace68/1
  reord_dvalid_delay2/1 -> [hmc_reord_dvalid]
  Gateway Out81/1 -> To Workspace75/1
  Gateway Out82/1 -> To Workspace76/1
  [hmc_reord_dvalid] -> FIFO1/2
  bus_expand1/1(msb_out8) -> pipeline37/1(d)  "hmc_out1"
  bus_expand1/8(lsb_out1) -> pipeline44/1(d)  "hmc_out8"
  pipeline51/1(q) -> bus_expand1/1(bus_in)
  bus_expand2/1(msb_out8) -> pipeline26/1(d)  "hmc_out9"
  bus_expand2/8(lsb_out1) -> pipeline36/1(d)  "hmc_out16"
  pipeline52/1(q) -> bus_expand2/1(bus_in)
  [fifo0_dout] -> pipeline52/1(d)
  [hmc_reord_dvalid] -> edge_detect14/1(in)
  [hmc_reord_sync] -> pipeline50/1(d)
  pipeline37/1(q) -> fifo1/1(in_d00)
  pipeline38/1(q) -> fifo1/2(in_d01)
  pipeline39/1(q) -> fifo1/3(in_d02)
  pipeline41/1(q) -> fifo1/5(in_d04)
  pipeline42/1(q) -> fifo1/6(in_d05)
  pipeline43/1(q) -> fifo1/7(in_d06)
  pipeline36/1(q) -> fifo0/8(in_d07)
  pipeline35/1(q) -> fifo0/7(in_d06)
  pipeline34/1(q) -> fifo0/6(in_d05)
  pipeline33/1(q) -> fifo0/5(in_d04)
  pipeline32/1(q) -> fifo0/4(in_d03)
  pipeline31/1(q) -> fifo0/3(in_d02)
  pipeline30/1(q) -> fifo0/2(in_d01)
  pipeline26/1(q) -> fifo0/1(in_d00)
  bus_expand1/2(out7) -> pipeline38/1(d)
  bus_expand1/4(out5) -> pipeline40/1(d)
  bus_expand1/7(out2) -> pipeline43/1(d)
  bus_expand1/3(out6) -> pipeline39/1(d)
  bus_expand2/7(out2) -> pipeline35/1(d)
  bus_expand1/5(out4) -> pipeline41/1(d)
  bus_expand1/6(out3) -> pipeline42/1(d)
  bus_expand2/5(out4) -> pipeline33/1(d)
  bus_expand2/4(out5) -> pipeline32/1(d)
  bus_expand2/6(out3) -> pipeline34/1(d)
  bus_expand2/3(out6) -> pipeline31/1(d)
  bus_expand2/2(out7) -> pipeline30/1(d)
  pipeline49/1(q) -> pipeline45/1(d)
  [sync_trig] -> Logical10/2
  Logical10/1 -> pipeline46/1(d)
  sync_en_fifo/1(in_reg) -> pipeline54/1(d), pipeline48/1(d)
  pipeline48/1(q) -> Logical12/2
  pipeline50/1(q) -> Logical12/1
  Logical12/1 -> edge_detect9/1(in)
  pipeline44/1(q) -> fifo1/8(in_d07)
  pipeline40/1(q) -> fifo1/4(in_d03)
  edge_detect9/1(out) -> Logical10/1
  pipeline53/1(q) -> pipeline57/1(d)
  [sync_trig] -> Logical13/2
  edge_detect8/1(out) -> Logical13/1
  Logical13/1 -> pipeline56/1(d)
  Logical14/1 -> edge_detect8/1(in)
  pipeline54/1(q) -> Logical14/2
  pipeline55/1(q) -> Logical14/1
  [hmc_reord_sync] -> pipeline55/1(d)
  [hmc_reord_dvalid] -> edge_detect13/1(in)
  pipeline56/1(q) -> fifo0/14(trig)
  pipeline57/1(q) -> fifo0/13(we)
  [fifo1_dout] -> pipeline51/1(d)
  pipeline59/1(q) -> fifo0/10(in_per_full)
  pipeline58/1(q) -> fifo0/11(in_full)
  pipeline60/1(q) -> fifo0/9(in_empty)
  FIFO0/3 -> [fifo0_per_full]
  [fifo0_per_full] -> cd_hmc_fifo0_level/1(out_level)
  [fifo0_empty] -> pipeline62/1(d)
  [fifo0_full] -> pipeline64/1(d)
  [fifo0_per_full] -> pipeline63/1(d)
  pipeline62/1(q) -> pipeline60/1(d)
  pipeline63/1(q) -> pipeline59/1(d)
  pipeline64/1(q) -> pipeline58/1(d)
  FIFO1/3 -> [fifo1_per_full]
  [fifo1_per_full] -> cd_hmc_fifo1_level/1(out_level)
  FIFO0/1 -> [fifo0_dout]
  [fifo0_dout] -> bus_expand12/1(bus_in)
  FIFO1/1 -> [fifo1_dout]
  [fifo1_dout] -> bus_expand11/1(bus_in)
  [mux_sel] -> Gateway Out88/1, Mux/1
  edge_detect13/1(out) -> pipeline53/1(d)
  pipeline45/1(q) -> fifo1/13(we)
  pipeline46/1(q) -> fifo1/14(trig)
  pipeline65/1(q) -> fifo1/9(in_empty)
  pipeline66/1(q) -> fifo1/10(in_per_full)
  pipeline67/1(q) -> fifo1/11(in_full)
  pipeline68/1(q) -> pipeline67/1(d)
  pipeline69/1(q) -> pipeline66/1(d)
  pipeline70/1(q) -> pipeline65/1(d)
  [fifo1_empty] -> pipeline70/1(d)
  [fifo1_per_full] -> pipeline69/1(d)
  [fifo1_full] -> pipeline68/1(d)
  edge_detect14/1(out) -> pipeline49/1(d)
  pipeline71/1(q) -> pipeline72/1(d)
  pipeline72/1(q) -> fifo0/12(in_mux_sel)
  pipeline73/1(q) -> fifo1/12(in_mux_sel)
  pipeline74/1(q) -> pipeline73/1(d)
  [mux_sel] -> pipeline74/1(d)
  [mux_sel] -> pipeline71/1(d)
  bus_expand3/1(msb_out8) -> pipeline83/1(d)  "hmc_out1"
  bus_expand3/8(lsb_out1) -> pipeline90/1(d)  "hmc_out8"
  pipeline96/1(q) -> bus_expand3/1(bus_in)
  [q_dvalid] -> pipeline94/1(d)
  [q_sync] -> pipeline95/1(d)
  pipeline83/1(q) -> qout/1(in_d00)
  pipeline84/1(q) -> qout/2(in_d01)
  pipeline85/1(q) -> qout/3(in_d02)
  pipeline87/1(q) -> qout/5(in_d04)
  pipeline88/1(q) -> qout/6(in_d05)
  pipeline89/1(q) -> qout/7(in_d06)
  pipeline91/1(q) -> qout/11(we)
  pipeline92/1(q) -> qout/12(trig)
  bus_expand3/2(out7) -> pipeline84/1(d)
  bus_expand3/4(out5) -> pipeline86/1(d)
  bus_expand3/7(out2) -> pipeline89/1(d)
  bus_expand3/3(out6) -> pipeline85/1(d)
  bus_expand3/5(out4) -> pipeline87/1(d)
  bus_expand3/6(out3) -> pipeline88/1(d)
  pipeline94/1(q) -> pipeline91/1(d)
  [sync_trig] -> Logical15/2
  Logical15/1 -> pipeline92/1(d)
  sync_en_qout/1(in_reg) -> pipeline93/1(d)
  pipeline93/1(q) -> Logical16/2
  pipeline95/1(q) -> Logical16/1
  Logical16/1 -> edge_detect16/1(in)
  pipeline90/1(q) -> qout/8(in_d07)
  pipeline86/1(q) -> qout/4(in_d03)
  edge_detect16/1(out) -> Logical15/1
  [q_out] -> pipeline96/1(d)
  pipeline75/1(q) -> qout/9(in_dvalid)
  pipeline76/1(q) -> qout/10(in_sync)
  pipeline77/1(q) -> pipeline76/1(d)
  pipeline78/1(q) -> pipeline75/1(d)
  [q_dvalid] -> pipeline78/1(d)
  [q_sync] -> pipeline77/1(d)
  [hmc_reord_dvalid] -> FIFO0/2
  [fifo0_empty] -> Logical18/1
  [fifo1_empty] -> Logical18/2
  Logical18/1 -> edge_detect11/1(in), Delay7/1
  Delay7/1 -> Counter/2
  edge_detect11/1(out) -> Counter/1
  [fifo0_re] -> Inverter3/1
  Gateway Out88/1 -> To Workspace82/1
  [fifo0_dout] -> Mux/2
  [fifo1_dout] -> Mux/3
  [fifo1_re] -> Logical20/1
  Logical20/1 -> delay1/1
  Inverter3/1 -> Logical20/2
  Counter/1 -> Convert15/1, Convert14/1
  Inverter1/1 -> Logical21/1
  [fifo0_empty] -> Inverter7/1
  Logical21/1 -> [fifo0_re]
  Logical23/1 -> [fifo1_re]
  [fifo1_empty] -> Inverter8/1
  Inverter7/1 -> Logical21/2
  Inverter8/1 -> Logical23/2
  [fifo0_re] -> FIFO0/3
  [fifo1_re] -> FIFO1/3
  Convert14/1 -> Inverter1/1
  Convert15/1 -> Logical23/1
  delay1/1 -> [mux_sel]
  [mux_sel] -> edge_detect15/1(in)
  edge_detect15/1(out) -> delay3/1
  pipeline79/1(q) -> dv/1, Gateway Out21/1, [q_dvalid]
  delay3/1 -> pipeline79/1(d)
  pipeline113/1(q) -> Terminator/1
